simulink model "base"  (Simulink 6.1)
settings: Solver=FixedStepDiscrete  StartTime=0.0  StopTime=inf  FixedStep=0.001  RelTol=1e-3
PostLoadFcn:
  | ,try, rti_mdl_postloadfcn(bdroot, 'UpdateModel', 160, 'rti1005'); catch, disp(lasterr); end,
libraries: rtican x2, rtilibm x1, dsextras x1
settings Model: LastModifiedBy=yamakawa  ProdHWDeviceType=Specified
settings OptimizationCC: BlockReduction=off
settings DebuggingCC: SolverPrmCheckMsg=warning
settings HardwareCC: ProdIntDivRoundTo=Zero  ProdEndianess=BigEndian  ProdHWDeviceType=Specified  TargetIntDivRoundTo=Zero  TargetEndianess=BigEndian
settings RTWCC: SystemTargetFile=rti1005.tlc  MakeCommand=make_rti  TemplateMakefile=rti1005.tmf  Description=dSPACE DS1005 Hardware Platform  ProcessScript=rti1005_make_rtw_hook
settings STFCustomTargetCC: TargetFcnLib=ansi_tfl_tmw.mat  GenFloatMathFcnCalls=ANSI_C  ModelReferenceCompliant=off  SystemTargetFile=rti1005.tlc
settings GRTTargetCC: ModelReferenceCompliant=off  MatFileLogging=off  ExtModeMexFile=rti_comm
settings CustomProperty: DataType=RTWOptions_EnumType_c__dspace_matlab_rti1005_tlc_rti1005_InitialSimState  Value=STOP
settings EnumStrPairs: String=RUN

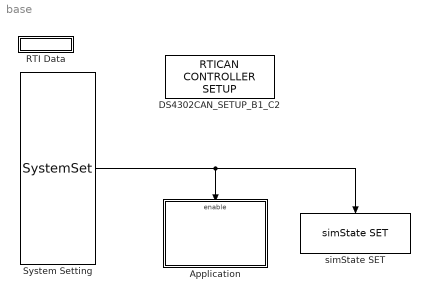
== system base ==
  Application : Subsystem  TreatAsAtomicUnit=on
  DS4302CAN_SETUP_B1_C2 : rtican/RTICAN CONTROLLER SETUP   Reserved1=[]  Reserved2=[]  Reserved3=[]  Reserved4=[]  AcceptanceMask=[]  ArbitrationField=[]  Parameters=[]  SFcnRTICANSettings=[]  MS_Struct=[]  BoardTypeNo=[]  BoardNo=[]  ChannelNo=[]  DialogFcn=[]  UnitName=[]  Revision=[]  UnitValues=[]  DSProperties=struct('RTI',struct('Version',uint32(7),'BlockType',struct('isSLSource',uint8(0),'isSLSink',uint8(0),'isHWSource',uint8(0),'isHWSink',uint8(0),'isSetup',uint8(1),'isInline',uint8(1),'isNonInline',uint8(0),'isInterrupt',uint8(0),'isChannelwise',uint8(0)),'IOBoardType','RTICAN','UnitType','NON_MESSAGE','Identifier','MASTER','DialogType','ML','BlockSet','RTICAN','SlaveProcessor','CAN'))  RTIBlockInterface=struct('InputPortsWidth',int32(0),'InputPortsActive',0,'OutputPortsWidth',int32(0),'OutputPortsActive',0,'DialogFcn','rtican_master_setup_gui','BlockDisplay',{{['CAN CONTROLLER\n SETUP'],'center'}},'IconTransparency','on','InitLevel',3,'IWork',{{{'',uint32(2)}}},'BlockName',struct('Token',{{'DS','CAN_SETUP_B','_C'}},'BlockParam',{{'BoardTypeNo','BoardNo','ChannelNo'}}),'ParameterTunableNames',{{}})  RTIBlockParameters=struct('BoardTypeNo',{{4302,'OFF',[]}},'BoardNo',{{1,'ON',[1 16]}},'ChannelNo',{{2,'ON',[1 4]}},'AcceptanceMask',{{0,'OFF',[]}},'ArbitrationField',{{0,'OFF',[]}},'Parameters',{{struct('Config',struct('Baudrate',500,'SampleMode',1,'UsedParamSet',1,'Standard',struct('Frequency',[16000000 16000000],'BTR0',[64 64],'BTR1',[28 28],'isBTRvalues',0,'Settings',struct('SMPL',[0 0],'BRP',[0 0],'NBT',[16 16],'TSEG1',[12 12],'TSEG2',[1 1],'SJW',[1 1],'SP',[87 87]),'validSettings',1),'Alternative',struct('Frequency',[16000000 16000000],'BTR0',[64 64],'BTR1',[28 28],'isBTRvalues',0,'Settings',struct('SMPL',[0 0],'BRP',[0 0],'NBT',[16 16],'TSEG1',[12 12],'TSEG2',[1 1],'SJW',[1 1],'SP',[87 87]),'validSettings',1)),'configType',1,'Options',struct('DataFileSelected',0,'DataFileName',{{['<no datafile support>']}},'DataFileDate',{{''}},'InterfaceFcn','rtican_dbc_file_parser','InterfaceFcnFileName','','LabelConfigType','volatile','AcceptanceMaskSelected',0,'MsgDataType','AllwaysDouble','NumType','hex','MaskType','STD','AcceptanceMask',0,'ArbitrationField',0,'UseMultipleMessageAccess',0),'RxReceiveStdOptions',struct('RxServiceStdEnabled',0,'RxServiceStdMsgIdent',1000,'RxServiceStdIdentNumType',1,'RxServiceStdIdentMask',0,'RxServiceStdMaskNumType',1,'RxServiceStdQueueSize',64),'RxReceiveXtdOptions',struct('RxServiceXtdEnabled',0,'RxServiceXtdMsgIdent',1001,'RxServiceXtdIdentNumType',1,'RxServiceXtdIdentMask',0,'RxServiceXtdMaskNumType',1,'RxServiceXtdQueueSize',64),'general',struct('Termination_common',1,'Termination_C252',1,'BusConfigurationRegister',0,'Transceiver','ISO11898','isFromLib',0)),'OFF',[]}},'CCPParameters',{{struct('CRO',struct('Format','STD','NumFormat','hex','Id',1639),'DTO',struct('Format','STD','NumFormat','hex','Id',2017),'StationAdr',struct('NumFormat','hex','Value',57),'StationId',struct('Value',['dSPACE CCP Service']),'Enabled',0),'OFF',[]}},'GroupId',{{struct('Group',{{'RTICAN'}},'No',1,'Behavior',{{'EVER'}},'BlockType',{{'SOURCE'}},'NameChangeFlag',1),'OFF',[]}},'SFcnRTICANSettings',{{struct('Baudrate',500,'Frequency',16000000,'BitTiming0','0x40','BitTiming1','0x1C','alterFrequency',16000000,'alterBitTmg0','0x40','alterBitTmg1','0x1C','UsedParamSet',1,'STDMaskSelected','no','XTDMaskSelected','no','BoardType','DS4302','BoardNo',1,'ControllerNo',2,'Transceiver','ISO11898','BusConfigRegister',0,'TerminationRes',120,'UseMultipleMessageAccess','no','STDRXSrvcUsed','no','STDRXSrvcMsgId',1000,'STDRXSrvcMsgMask',0,'STDRXSrvcQueueSize',64,'XTDRXSrvcUsed','no','XTDRXSrvcMsgId',1001,'XTDRXSrvcQueueSize',64,'XTDRXSrvcMsgMask',0),'OFF',[]}},'SFcnRTICCPSettings',{{struct('CRO',struct('Format','STD','NumFormat','hex','Id',1639),'DTO',struct('Format','STD','NumFormat','hex','Id',2017),'StationAdr',struct('NumFormat','hex','Value',57),'StationId',struct('Value',['dSPACE CCP Service']),'Enabled',0),'OFF',[]}},'TLCFileName',{{'rtican_master_setup','OFF',[]}})  RTISFcnParameters=struct('SFcnRTICANSettings','struct','SFcnRTICCPSettings','struct','AcceptanceMask','int32','ArbitrationField','int32','TLCFileName','char')  RTIBlockParaDefault=struct('BoardTypeNo',4302,'BoardNo',1,'ChannelNo',1,'AcceptanceMask',0,'ArbitrationField',0,'Parameters',struct('Config',struct('Baudrate',500,'SampleMode',1,'UsedParamSet',1,'Standard',struct('Frequency',[16000000 16000000],'BTR0',[64 64],'BTR1',[28 28],'isBTRvalues',0,'Settings',struct('SMPL',[0 0],'BRP',[0 0],'NBT',[16 16],'TSEG1',[12 12],'TSEG2',[1 1],'SJW',[1 1],'SP',[87 87]),'validSettings',1),'Alternative',struct('Frequency',[16000000 16000000],'BTR0',[64 64],'BTR1',[28 28],'isBTRvalues',0,'Settings',struct('SMPL',[0 0],'BRP',[0 0],'NBT',[16 16],'TSEG1',[12 12],'TSEG2',[1 1],'SJW',[1 1],'SP',[87 87]),'validSettings',1)),'configType',1,'Options',struct('DataFileSelected',0,'DataFileName',{{['<no datafile support>']}},'DataFileDate',{{''}},'InterfaceFcn','rtican_dbc_file_parser','InterfaceFcnFileName','','LabelConfigType','volatile','AcceptanceMaskSelected',0,'MsgDataType','AllwaysDouble','NumType','hex','MaskType','STD','AcceptanceMask',0,'ArbitrationField',0,'UseMultipleMessageAccess',0),'RxReceiveStdOptions',struct('RxServiceStdEnabled',0,'RxServiceStdMsgIdent',1000,'RxServiceStdIdentNumType',1,'RxServiceStdIdentMask',0,'RxServiceStdMaskNumType',1,'RxServiceStdQueueSize',64),'RxReceiveXtdOptions',struct('RxServiceXtdEnabled',0,'RxServiceXtdMsgIdent',1001,'RxServiceXtdIdentNumType',1,'RxServiceXtdIdentMask',0,'RxServiceXtdMaskNumType',1,'RxServiceXtdQueueSize',64),'general',struct('Termination_common',1,'Termination_C252',1,'BusConfigurationRegister',0,'Transceiver','ISO11898','isFromLib',1)),'CCPParameters',struct('CRO',struct('Format','STD','NumFormat','hex','Id',1639),'DTO',struct('Format','STD','NumFormat','hex','Id',2017),'StationAdr',struct('NumFormat','hex','Value',57),'StationId',struct('Value',['dSPACE CCP Service']),'Enabled',0),'GroupId',struct('Group',{{'RTICAN'}},'No',1,'Behavior',{{'EVER'}},'BlockType',{{'SOURCE'}},'NameChangeFlag',1),'SFcnRTICANSettings',struct('Baudrate',500,'Frequency',16000000,'BitTiming0','0x40','BitTiming1','0x1C','alterFrequency',36000000,'alterBitTiming0','0x40','alterBitTiming1','0x1C','UsedParamSet',1,'STDMaskSelected','no','XTDMaskSelected','no','BoardType','DS4302','BoardNo',1,'ControllerNo',1,'Transceiver','ISO11898','BusConfigRegister',0,'TerminationRes',120,'UseMultipleMessageAccess','no','STDRXSrvcUsed','no','STDRXSrvcMsgId',1000,'STDRXSrvcMsgMask',0,'STDRXSrvcQueueSize',64,'XTDRXSrvcUsed','no','XTDRXSrvcMsgId',1001,'XTDRXSrvcQueueSize',64,'XTDRXSrvcMsgMask',0),'SFcnRTICCPSettings',struct('CRO',struct('Format','STD','NumFormat','hex','Id',1639),'DTO',struct('Format','STD','NumFormat','hex','Id',2017),'StationAdr',struct('NumFormat','hex','Value',57),'StationId',struct('Value',['dSPACE CCP Service']),'Enabled',0),'TLCFileName','rtican_master_setup')
      settings: AttributesFormatString=Group Id: RTICAN1\n
  RTI Data : Subsystem  Tag=struct('RTIDataServer',struct('RTIDataServerVs','2','RTIModelDescription','struct(''main'',''base'',''sub'','''',''isMp'',0)'))  LoadFcn="if exist('rtidc'), try,  rtidc('DataHostBlockClbLoad', gcbh); catch, disp(['Warning: ''LoadFcn'' for RTI Data block failed: ' lasterr]); end, end,"
      settings: CopyFcn="if exist('rtidc'), try,  rtidc('DataHostBlockClbCopy', gcbh); catch, disp(['Warning: ''CopyFcn'' for RTI Data block failed: ' lasterr]); end, end,"  DeleteFcn="if exist('rtidc'), try,  rtidc('DataHostBlockClbDelete', gcbh); catch, disp(['Warning: ''DeleteFcn'' for RTI Data block failed: ' lasterr]); end, end,"  ModelCloseFcn="if exist('rtidc'), try,  rtidc('DataHostBlockClbModelClose', gcbh); catch, disp(['Warning: ''ModelCloseFcn'' for RTI Data block failed: ' lasterr]); end, end,"  PreSaveFcn="if exist('rtidc'), try,  rtidc('DataHostBlockClbPreSave', gcbh); catch, disp(['Warning: ''PreSaveFcn'' for RTI Data block failed: ' lasterr]); end, end,"  PostSaveFcn="if exist('rtidc'), try,  rtidc('DataHostBlockClbPostSave', gcbh); catch, disp(['Warning: ''PostSaveFcn'' for RTI Data block failed: ' lasterr]); end, end,"  NameChangeFcn="if exist('rtidc'), try,  rtidc('DataHostBlockClbNameChange', gcbh); catch, disp(['Warning: ''NameChangeFcn'' for RTI Data block failed: ' lasterr]); end, end,"
      mask Type: RTI_DATA_HOST
      mask Description:
      | RTI Data Block.
      | This block is used by RTI to store internal model-dependent data.
      | Please keep this block on the root level of the model. Deleting this block will result in data loss.
      | 
      | NEVER DELETE OR COPY THIS BLOCK!
      mask Help:
      | RTI Data Block.
      | This block is used by RTI to store internal model-dependent data.
      | Please keep this block on the root level of the model. Deleting this block will result in data loss.
      | 
      | NEVER DELETE OR COPY THIS BLOCK!
      mask Display:
      | text(0.5, 0.5, 'RTI Data', 'HorizontalAlignment', 'center');
      | plot([1 0]);
  System Setting : S-Function  FunctionName=SystemSet
  simState SET : dsextras/simState SET  TriggerPort=falling  EnablePort=none  SimStateMode=STOP  TLCFileName=rti_simstate_set  Reserved1=[]  Reserved2=[]  Reserved3=[]  Reserved4=[]  DSProperties=struct('RTI',struct('Version',uint32(1),'BlockType',struct('isSLSource',uint8(1),'isSLSink',uint8(0),'isHWSource',uint8(0),'isHWSink',uint8(0),'isSetup',uint8(0),'isInline',uint8(1),'isNonInline',uint8(0),'isInterrupt',uint8(0),'isChannelwise',uint8(0)),'IOBoardType','EXTRAS','UnitType','SIMSTATESET','Identifier','SIMSTATESET','DialogType','SL','BlockSet','NONE','SlaveProcessor','NONE'))  RTIBlockInterface=struct('OutputPortsWidth',int32(0),'BlockDisplay',{{['simState STOP'],'center'}},'IconTransparency','on','InitLevel',2,'BlockName',struct('Token',{{['simState SET']}}),'TriggerPort',{{'falling'}},'EnablePort',{{'none'}},'MaskDescription',['Set simState to the specified value when the block is executed.'])  RTIBlockParameters=struct('TriggerPort',{{3,'OFF',[]}},'EnablePort',{{1,'OFF',[]}},'SimStateMode',{{3,'OFF',[]}},'TLCFileName',{{'rti_simstate_set','OFF',[]}})  RTISFcnParameters=struct('TriggerPort','double','EnablePort','double','SimStateMode','char','TLCFileName','char')  RTIBlockParaDefault=struct('TriggerPort',2,'EnablePort',1,'SimStateMode',1,'TLCFileName','rti_simstate_set')
  wires:
  System Setting/1 -> Application/Enable, simState SET/Trigger

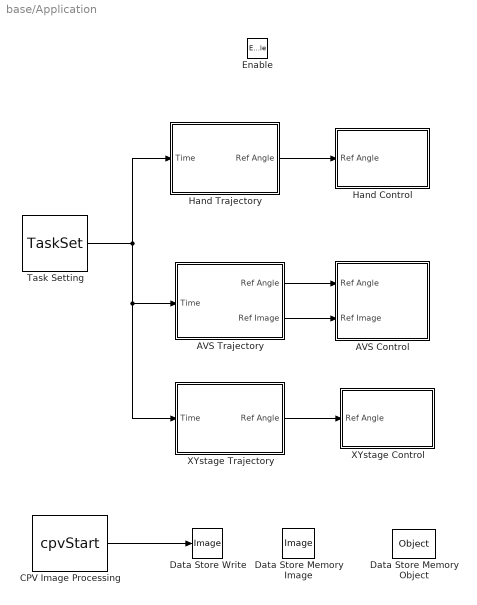
== system base/Application ==
  Enable : EnablePort  StatesWhenEnabling=reset
  AVS Control : Subsystem
  AVS Trajectory : Subsystem
  CPV Image Processing : S-Function  FunctionName=cpvStart
  Data Store Write : DataStoreWrite  DialogController=Simulink.DDGSource  DataStoreName=Image  SampleTime=-1
  Data Store Memory Image : DataStoreMemory  DialogController=Simulink.DDGSource  DataStoreName=Image  InitialValue=[-1 -1 0 0 0 0 0 0 0 0 0 0 0 0 0 0]  DataType=double
  Data Store Memory Object : DataStoreMemory  DialogController=Simulink.DDGSource  DataStoreName=Object  InitialValue=[-1 0 0 0 0 0 0 0 0 0 0 0 0 0 0 0]  DataType=double
  Hand Control : Subsystem
  Hand Trajectory : Subsystem
  Task Setting : S-Function  FunctionName=TaskSet
  XYstage Control : Subsystem
  XYstage Trajectory : Subsystem
  wires:
  Hand Trajectory/1(Ref Angle) -> Hand Control/1(Ref Angle)
  AVS Trajectory/1(Ref Angle) -> AVS Control/1(Ref Angle)
  Task Setting/1 -> Hand Trajectory/1(Time), AVS Trajectory/1(Time), XYstage Trajectory/1(Time)
  AVS Trajectory/2(Ref Image) -> AVS Control/2(Ref Image)
  CPV Image Processing/1 -> Data Store Write/1
  XYstage Trajectory/1(Ref Angle) -> XYstage Control/1(Ref Angle)

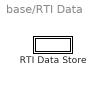
== system base/RTI Data ==
  RTI Data Store : Subsystem  Tag="struct('private',struct('version',struct('dsVer',uint32(2),'dsVerCreation',uint32(2),'RTI',struct('ver','5.2.5','type','RTI1005')),'access',struct('type','Model','isPerm',1,'created',['11-Nov-2005 16:55:46'],'modified',['16-May-2008 17:11:14'],'location','')),'public',struct('main',struct('data',[]),'sub',struct('name',{{'base'}},'data',{{struct('TH',struct('thTaskInfo',struct('taskType',{'TIMER','HWINT','TMRINT','SWINT'},'tasksNumOf',{1,0,0,0},'srcIds',{{'TIMERA'},{},{},{}},'taskNames',{{['Timer Task 1']},{},{},{}})),'th_tc',struct('dataType','TASK','taskGroupId','','taskGroupList',{{}},'taskSchedulingPolicy','FCFS','taskType','TIMER','blkh',-1,'srcId','TIMERA','srcSgnName',['Timer A interrupt'],'srcCpuName','','taskName',['Timer Task 1  [0.001] s'],'taskNameDisplayExt','','smplTime',0.001,'smplTimeOffs',0,'hasFixedPriority',0,'priority',1,'hasFixedOvc',0,'ovcType',1,'ovcMax',1),'tc_th',struct('dataType','TASK','taskGroupId','','taskGroupList',{{}},'taskSchedulingPolicy','FCFS','taskType','TIMER','blkh',-1,'srcId','TIMERA','srcSgnName',['Timer A interrupt'],'srcCpuName','','taskName',['Timer Task 1  [0.001] s'],'taskNameDisplayExt','','smplTime',0.001,'smplTimeOffs',0,'hasFixedPriority',0,'priority',1,'hasFixedOvc',0,'ovcType',1,'ovcMax',1))}})))"
      mask Type: RTI_DATA_STORE
      mask Description:
      | RTI Data Store Block. This block is used by RTI to store internal model dependent data. Deleting this block will result in data loss.
      | 
      | NEVER DELETE, COPY, OR MODIFY THIS BLOCK!
      mask Help:
      | RTI Data Store Block. This block is used by RTI to store internal model dependent data. Deleting this block will result in data loss.
      | 
      | NEVER DELETE, COPY, OR MODIFY THIS BLOCK!
      mask Display: text(0.5, 0.5, ' ', 'HorizontalAlignment', 'center');

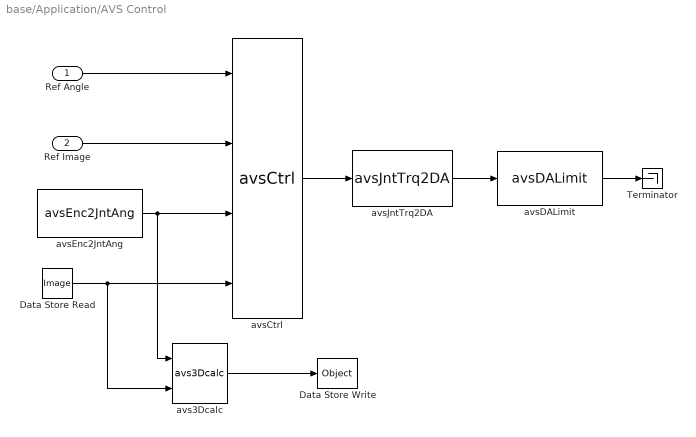
== system base/Application/AVS Control ==
  Ref Angle : Inport  Port=1  LatchInput=off
  Ref Image : Inport  Port=2  LatchInput=off
  Data Store Read : DataStoreRead  DialogController=Simulink.DDGSource  DataStoreName=Image  SampleTime=0
  Data Store Write : DataStoreWrite  DialogController=Simulink.DDGSource  DataStoreName=Object  SampleTime=-1
  Terminator : Terminator
  avs3Dcalc : S-Function  FunctionName=avs3Dcalc
  avsCtrl : S-Function  FunctionName=avsCtrl
  avsDALimit : S-Function  FunctionName=avsDALimit
  avsEnc2JntAng : S-Function  FunctionName=avsEnc2JntAng
  avsJntTrq2DA : S-Function  FunctionName=avsJntTrq2DA
  wires:
  Ref Angle/1 -> avsCtrl/1
  avsCtrl/1 -> avsJntTrq2DA/1
  avsJntTrq2DA/1 -> avsDALimit/1
  avsDALimit/1 -> Terminator/1
  Ref Image/1 -> avsCtrl/2
  avsEnc2JntAng/1 -> avsCtrl/3, avs3Dcalc/1
  Data Store Read/1 -> avsCtrl/4, avs3Dcalc/2
  avs3Dcalc/1 -> Data Store Write/1

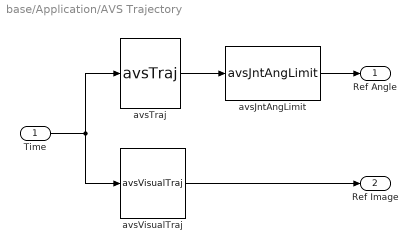
== system base/Application/AVS Trajectory ==
  Time : Inport  Port=1  LatchInput=off
  avsJntAngLimit : S-Function  FunctionName=avsJntAngLimit
  avsTraj : S-Function  FunctionName=avsTraj
  avsVisualTraj : S-Function  FunctionName=avsVisualTraj
  Ref Angle : Outport
  Ref Image : Outport  Port=2
  wires:
  Time/1 -> avsTraj/1, avsVisualTraj/1
  avsTraj/1 -> avsJntAngLimit/1
  avsJntAngLimit/1 -> Ref Angle/1
  avsVisualTraj/1 -> Ref Image/1

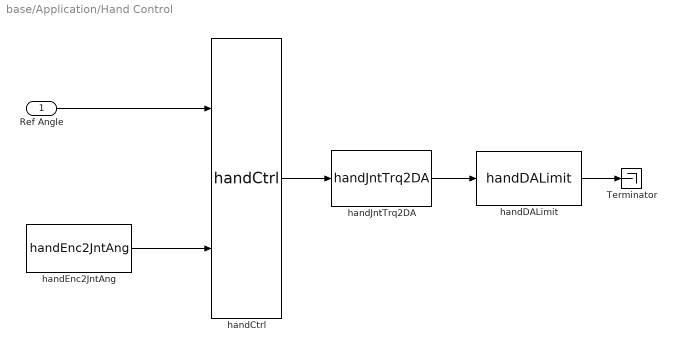
== system base/Application/Hand Control ==
  Ref Angle : Inport  Port=1  LatchInput=off
  Terminator : Terminator
  handCtrl : S-Function  FunctionName=handCtrl
  handDALimit : S-Function  FunctionName=handDALimit
  handEnc2JntAng : S-Function  FunctionName=handEnc2JntAng
  handJntTrq2DA : S-Function  FunctionName=handJntTrq2DA
  wires:
  Ref Angle/1 -> handCtrl/1
  handEnc2JntAng/1 -> handCtrl/2
  handCtrl/1 -> handJntTrq2DA/1
  handJntTrq2DA/1 -> handDALimit/1
  handDALimit/1 -> Terminator/1

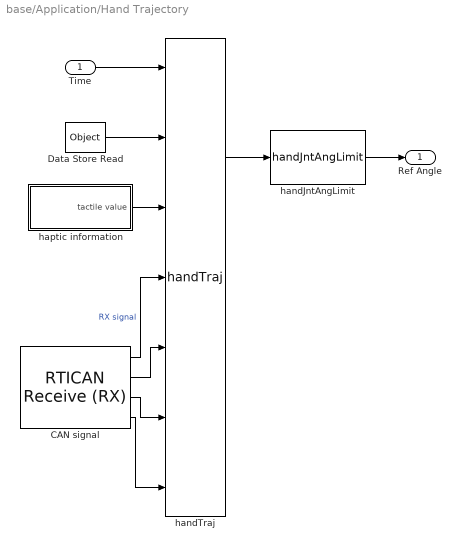
== system base/Application/Hand Trajectory ==
  Time : Inport  Port=1  LatchInput=off
  CAN signal : rtican/RTICAN Receive (RX)   Reserved1=[]  Reserved2=[]  Reserved3=[]  Reserved4=[]  SfcnMessage=[]  Msg_Struct=[]  BoardTypeNo=[]  BoardNo=[]  ChannelNo=[]  Parameters=[]  DialogFcn=[]  UnitName=[]  Revision=[]  UnitValues=[]  DSProperties=struct('RTI',struct('Version',uint32(5),'BlockType',struct('isSLSource',uint8(1),'isSLSink',uint8(1),'isHWSource',uint8(0),'isHWSink',uint8(0),'isSetup',uint8(0),'isInline',uint8(1),'isNonInline',uint8(0),'isInterrupt',uint8(0),'isChannelwise',uint8(0)),'IOBoardType','RTICAN','UnitType','MESSAGE','Identifier','RX','DialogType','MSVC','BlockSet','RTICAN','SlaveProcessor','CAN'))  RTIBlockInterface=struct('OutputPortsWidth',int32([1 1 1 1]),'OutputPortsActive',[1 1 1 1],'OutputPortsName',{{['RX signal'],['RX status'],['RX time'],['RX delta time']}},'OutputPortsDataType',{{'SS_DOUBLE','SS_DOUBLE','SS_DOUBLE','SS_DOUBLE'}},'OutputPortsLabel',{{['RX signal'],'','',''}},'OutputPortsLabelMode','ON','InputPortsWidth',int32(0),'InputPortsActive',0,'DialogFcn','rtican_message_interface_gui','BlockDisplay',{{'','center'}},'IconTransparency','on','ParameterTunableNames',{{}},'InitLevel',3,'BlockName',struct('Token',{{'DS','CAN_RX_B','_C'}},'BlockParam',{{'BoardTypeNo','BoardNo','ChannelNo'}}),'SampleTime',{{-1}},'TriggerPort',{{'none'}},'EnablePort',{{'none'}})  RTIBlockParameters=struct('BoardTypeNo',{{4302,'OFF',[]}},'BoardNo',{{1,'ON',[1 16]}},'ChannelNo',{{2,'ON',[1 4]}},'Parameters',{{struct('DataFileSupport',struct('DataFileSelectedMaster',0,'DataFileSelectedLocal',0,'DataFileName',['<no datafile support>|'],'DataFileDate','','SelectedFile',['<no file selected>']),'Options',struct('StatusSelected',1,'TimeSelected',1,'DeltaTimeSelected',1,'BytePortSelected',0,'MessageLengthSelected',0,'TriggerPort',struct('Selected',0,'TriggerType',0),'UserCoding',struct('Selected',0,'InterfaceFile','UserDecodingFile','FcnName','UserDecodeFcn','InportSelected',0,'InportWidth',1,'OutportSelected',0,'OutportWidth',1),'EnablePortSelected',0,'SignalOnPortnameSelected',1,'UseRXService',0),'Message',struct('MsgOnBlocknameSelected',1,'MsgName',['CAN signal'],'MsgIdFormat',0,'MsgId',0,'MsgLength',8,'NumSignals',1,'SampleTime',-1,'Signal',struct('SgnName',['RX signal'],'SgnStartBit',0,'SgnLength',8,'SgnType',0,'ModeValue',-1,'DataType',0,'ByteLayout',0,'Factor',1,'Offset',0,'SgnComment',{{''}},'SgnUnit','','Min',0,'Max',255,'SLDataType','SS_DOUBLE'),'MsgIdNumFormat',1,'MsgComment',{{''}}),'Version',1.2,'general',struct('isFromLib',0)),'OFF',[]}},'GroupId',{{struct('Group',{{'RTICAN'}},'No',1,'Behavior',{{'NAMECHANGE'}},'BlockType',{{'SINK'}},'NameChangeFlag',0),'OFF',[]}},'SFcnRTICANMessage',{{struct('MsgType','RX','SFcnPortType','Scalar','MsgName',['CAN signal'],'MsgIdFormat','STD','MsgId',0,'MsgLength',8,'NumSignals',1,'SampleTime',-1,'Signal',struct('SgnName',['RX signal'],'SgnStartBit',0,'SgnLength',8,'SgnType','standard','ModeValue',-1,'DataType',['unsigned int'],'ByteLayout',['little endian'],'Factor',1,'Offset',0,'SLDataType','SS_DOUBLE'),'StatusSelected','yes','TimeSelected','yes','DeltaTimeSelected','yes','BytePortSelected','no','MessageLengthSelected','no','TriggerPort',struct('Selected','no','TriggerType',0),'UserCoding',struct('Selected','no','InterfaceFile','UserDecodingFile','FcnName','UserDecodeFcn','InportSelected','no','InportWidth',1,'OutportSelected','no','OutportWidth',1),'EnablePortSelected','no','UseRXService','no','BoardType','DS4302','BoardNo',1,'ControllerNo',2),'OFF',[]}},'TLCFileName',{{'rtican_rx_message','OFF',[]}})  RTISFcnParameters=struct('SFcnRTICANMessage','struct','TLCFileName','char')  RTIBlockParaDefault=struct('BoardTypeNo',4302,'BoardNo',1,'ChannelNo',1,'Parameters',struct('DataFileSupport',struct('DataFileSelectedMaster',0,'DataFileSelectedLocal',0,'DataFileName','','DataFileDate','','SelectedFile',['<no file selected>']),'Options',struct('StatusSelected',1,'TimeSelected',1,'DeltaTimeSelected',1,'BytePortSelected',0,'MessageLengthSelected',0,'TriggerPort',struct('Selected',0,'TriggerType','rising'),'UserCoding',struct('Selected',0,'InterfaceFile','UserDecodingFile','FcnName','UserDecodeFcn','InportSelected',0,'InportWidth',1,'OutportSelected',0,'OutportWidth',1),'EnablePortSelected',0,'SignalOnPortnameSelected',1,'UseRXService',0),'Message',struct('MsgOnBlocknameSelected',0,'MsgName',['RX Message'],'MsgIdFormat',0,'MsgId',100,'MsgLength',8,'NumSignals',1,'SampleTime',-1,'Signal',struct('SgnName',['RX signal'],'SgnStartBit',0,'SgnLength',8,'SgnType',0,'ModeValue',-1,'DataType',0,'SLDataType','SS_DOUBLE','ByteLayout',0,'Factor',1,'Offset',0,'Min',0,'Max',255,'SgnComment',{{}},'SgnUnit',''),'MsgIdNumFormat',0,'MsgComment',{{''}}),'Version',1.2,'general',struct('isFromLib',1)),'GroupId',struct('Group',{{'RTICAN'}},'No',1,'Behavior',{{'NAMECHANGE'}},'BlockType',{{'SINK'}},'NameChangeFlag',0),'SFcnRTICANMessage',struct('MsgType','RX','MsgName',['RX Message'],'MsgIdFormat','STD','MsgId',100,'MsgLength',8,'NumSignals',1,'SampleTime',-1,'Signal',struct('SgnName',['RX signal'],'SgnStartBit',0,'SgnLength',8,'SgnType','standard','ModeValue',-1,'DataType',['unsigned int'],'ByteLayout',['little endian'],'SLDataType','SS_DOUBLE','Factor',1,'Offset',0),'StatusSelected','yes','TimeSelected','yes','DeltaTimeSelected','yes','BytePortSelected','no','MessageLengthSelected','no','EnablePortSelected','no','UserCoding',struct('Selected','no','InterfaceFile','UserDecodingFile','FcnName','UserDecodeFcn','InportSelected','no','InportWidth',1,'OutportSelected','no','OutportWidth',1),'TriggerPort',struct('Selected','no','TriggerType','rising'),'UseRXService','no','BoardType','DS4302','BoardNo',1,'ControllerNo',1,'SFcnPortType','Scalar'),'TLCFileName','rtican_rx_message')
      settings: AttributesFormatString=Group Id: RTICAN1\n
  Data Store Read : DataStoreRead  DialogController=Simulink.DDGSource  DataStoreName=Object  SampleTime=0
  handJntAngLimit : S-Function  FunctionName=handJntAngLimit
  handTraj : S-Function  FunctionName=handTraj
  "haptic information " : Subsystem
  Ref Angle : Outport
  wires:
  handTraj/1 -> handJntAngLimit/1
  Time/1 -> handTraj/1
  handJntAngLimit/1 -> Ref Angle/1
  Data Store Read/1 -> handTraj/2
  "haptic information "/1(tactile value) -> handTraj/3
  CAN signal/1 -> handTraj/4  "RX signal"
  CAN signal/2 -> handTraj/5
  CAN signal/3 -> handTraj/6
  CAN signal/4 -> handTraj/7

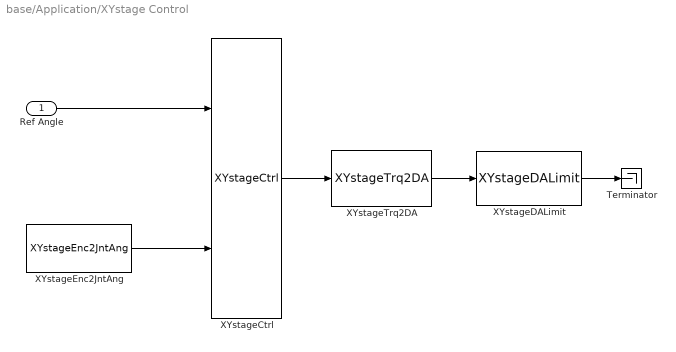
== system base/Application/XYstage Control ==
  Ref Angle : Inport  Port=1  LatchInput=off
  Terminator : Terminator
  XYstageCtrl : S-Function  FunctionName=XYstageCtrl
  XYstageDALimit : S-Function  FunctionName=XYstageDALimit
  XYstageEnc2JntAng : S-Function  FunctionName=XYstageEnc2JntAng
  XYstageTrq2DA : S-Function  FunctionName=XYstageTrq2DA
  wires:
  XYstageDALimit/1 -> Terminator/1
  XYstageTrq2DA/1 -> XYstageDALimit/1
  XYstageCtrl/1 -> XYstageTrq2DA/1
  XYstageEnc2JntAng/1 -> XYstageCtrl/2
  Ref Angle/1 -> XYstageCtrl/1

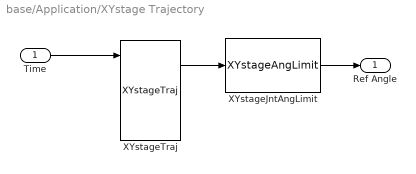
== system base/Application/XYstage Trajectory ==
  Time : Inport  Port=1  LatchInput=off
  XYstageJntAngLimit : S-Function  FunctionName=XYstageAngLimit
  XYstageTraj : S-Function  FunctionName=XYstageTraj
  Ref Angle : Outport
  wires:
  XYstageJntAngLimit/1 -> Ref Angle/1
  Time/1 -> XYstageTraj/1
  XYstageTraj/1 -> XYstageJntAngLimit/1

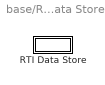
== system base/RTI Data/RTI Data Store ==
  RTI Data Store : Subsystem
      mask Type: RTI_DATA_STORE
      mask Description:
      | RTI Data Store Block. This block is used by RTI to store internal model dependent data. Deleting this block will result in data loss.
      | 
      | NEVER DELETE, COPY, OR MODIFY THIS BLOCK!
      mask Help:
      | RTI Data Store Block. This block is used by RTI to store internal model dependent data. Deleting this block will result in data loss.
      | 
      | NEVER DELETE, COPY, OR MODIFY THIS BLOCK!
      mask Display: text(0.5, 0.5, ' ', 'HorizontalAlignment', 'center');

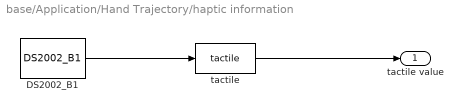
== system base/Application/Hand Trajectory/haptic information  ==
  DS2002_B1 : rtilibm/DS2002/DS2002_B1  BoardNo=1  ChannelNos=[1 2 3 4 5 6 7 8 9 10 11 12 13 14 15 16 17 18 19 20 21 22 23 24 25 26 27 28 29 30]  Range=[10 10]  Resolution=[16 16]  SampleAndHoldMode=[1 1]  DialogFcn=gui2002  UnitName={ 'DS2002_B' }  UnitValues={ 1 }  DSProperties=struct('RTI',struct('Version',uint32(1),'BlockType',struct('isSLSource',uint8(1),'isSLSink',uint8(0),'isHWSource',uint8(1),'isHWSink',uint8(0),'isSetup',uint8(0),'isInline',uint8(1),'isNonInline',uint8(0),'isInterrupt',uint8(0),'isChannelwise',uint8(0)),'IOBoardType','DS2002','UnitType','ADC','Identifier','ADCMUX','DialogType','ML','BlockSet','NONE','SlaveProcessor','NONE'))
  tactile : S-Function  FunctionName=tactile
  tactile value : Outport
  wires:
  tactile/1 -> tactile value/1
  DS2002_B1/1 -> tactile/1

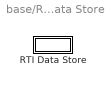
== system base/RTI Data/RTI Data Store/RTI Data Store ==
  RTI Data Store : Subsystem
      mask Type: RTI_DATA_STORE
      mask Description:
      | RTI Data Store Block. This block is used by RTI to store internal model dependent data. Deleting this block will result in data loss.
      | 
      | NEVER DELETE, COPY, OR MODIFY THIS BLOCK!
      mask Help:
      | RTI Data Store Block. This block is used by RTI to store internal model dependent data. Deleting this block will result in data loss.
      | 
      | NEVER DELETE, COPY, OR MODIFY THIS BLOCK!
      mask Display: text(0.5, 0.5, ' ', 'HorizontalAlignment', 'center');

== system base/RTI Data/RTI Data Store/RTI Data Store/RTI Data Store ==
  RTI Data Store : Subsystem
      mask Type: RTI_DATA_STORE
      mask Description:
      | RTI Data Store Block. This block is used by RTI to store internal model dependent data. Deleting this block will result in data loss.
      | 
      | NEVER DELETE, COPY, OR MODIFY THIS BLOCK!
      mask Help:
      | RTI Data Store Block. This block is used by RTI to store internal model dependent data. Deleting this block will result in data loss.
      | 
      | NEVER DELETE, COPY, OR MODIFY THIS BLOCK!
      mask Display: text(0.5, 0.5, ' ', 'HorizontalAlignment', 'center');

== system base/RTI Data/RTI Data Store/RTI Data Store/RTI Data Store/RTI Data Store ==
